simulink model "zigeler"  (R2025b)
settings: Solver=VariableStepAuto  StartTime=0.0  StopTime=10.0  RelTol=1e-3
values from neighbouring files (symbols this model uses):
  denW = W.Denominator{1}    [pid_ziegler.m]
  Kc = 10    [pid_ziegler.m]
  numW = W.Numerator{1}    [pid_ziegler.m]
settings Model: Creator=PROBOOK  LastModifiedBy=PROBOOK

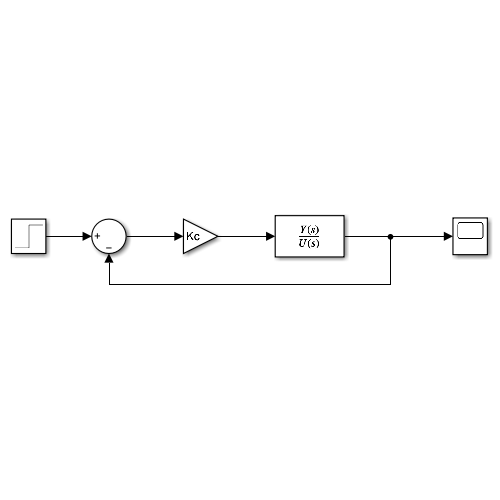
[thumbnail: Simulink's stored preview of the top-level diagram]
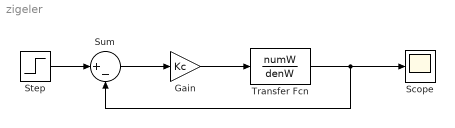
== system zigeler ==
  Gain : Gain  Gain=Kc
  Scope : Scope
      settings: ActiveDisplayYMinimum=-0.17130885649479635  ActiveDisplayYMaximum=1.5417797084531675
  Step : Step  SampleTime=0
  Sum : Sum  Inputs=|+-
  Transfer Fcn : TransferFcn  Numerator=numW  Denominator=denW
  wires:
  Sum/1 -> Gain/1
  Gain/1 -> Transfer Fcn/1
  Transfer Fcn/1 -> Sum/2, Scope/1
  Step/1 -> Sum/1
